simulink model "Batter_Model_02"  (Simulink 8.9)
settings: Solver=ode45  StartTime=0.0  StopTime=10.0  RelTol=1e-3  EnableMultiTasking=on
libraries: powerlib x2
settings Model: SuppressorTable=22 serialization::archive 11 0 6 0 0 0 0 0  Creator=hlopez5  LastModifiedBy=judithlopez
settings DataIOCC: SignalLoggingSaveFormat=Dataset
settings DebuggingCC: SolverPrmCheckMsg=warning  FcnCallInpInsideContextMsg=error
settings GRTTargetCC: CombineOutputUpdateFcns=on  GRTInterface=off

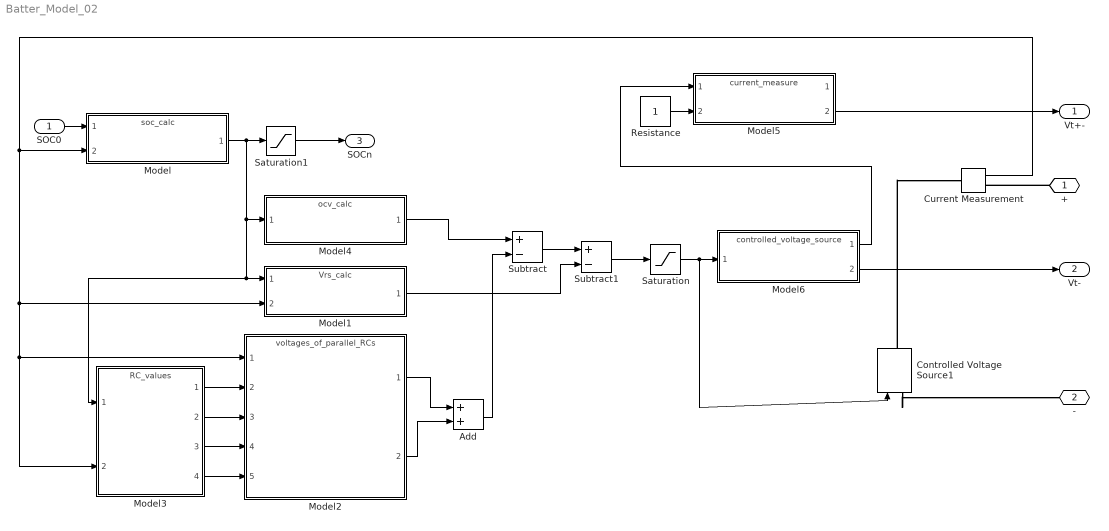
== system Batter_Model_02 ==
  SOC0 : Inport
  Add : Sum
  Controlled Voltage Source1 : powerlib/Electrical Sources/Controlled Voltage Source  Initialize=on  Source_Type=AC  Amplitude=0  Phase=0  Frequency=0  Measurements=None
  Current Measurement : powerlib/Measurements/Current Measurement  PhasorSimulation=off  OutputType=Complex  PSBequivalent=0
  Model : ModelReference  ModelNameDialog=soc_calc.mdl  SimulationMode=Normal  ModelReferenceVersion=1.2
  Model1 : ModelReference  ModelNameDialog=Vrs_calc.mdl  SimulationMode=Normal  ModelReferenceVersion=1.1
  Model2 : ModelReference  ModelNameDialog=voltages_of_parallel_RCs.mdl  SimulationMode=Normal  ModelReferenceVersion=1.3
  Model3 : ModelReference  ModelNameDialog=RC_values.mdl  SimulationMode=Normal  ModelReferenceVersion=1.3
  Model4 : ModelReference  ModelNameDialog=ocv_calc.mdl  SimulationMode=Normal  ModelReferenceVersion=1.1
  Model5 : ModelReference  ModelNameDialog=current_measure.mdl  SimulationMode=Normal  ModelReferenceVersion=1.3
  Model6 : ModelReference  ModelNameDialog=controlled_voltage_source.mdl  SimulationMode=Normal  ModelReferenceVersion=1.4
  Resistance : Constant
  Saturation : Saturate
  Saturation1 : Saturate
  Subtract : Sum  Inputs=+-
  Subtract1 : Sum  Inputs=+-
  " +" : PMIOPort  Port=1  Side=Left
  - : PMIOPort  Port=2  Side=Left
  Vt+- : Outport
  Vt- : Outport  Port=2
  SOCn : Outport  Port=3
  wires:
  Model3/1 -> Model2/2
  Model3/2 -> Model2/3
  Model3/3 -> Model2/4
  Model3/4 -> Model2/5
  Model2/1 -> Add/1
  Model2/2 -> Add/2
  Model4/1 -> Subtract/1
  Add/1 -> Subtract/2
  Subtract/1 -> Subtract1/1
  Model1/1 -> Subtract1/2
  Subtract1/1 -> Saturation/1
  SOC0/1 -> Model/1
  Model/1 -> Model3/1, Model1/1, Model4/1, Saturation1/1
  Saturation1/1 -> SOCn/1
  Current Measurement/1 -> Model3/2, Model2/1, Model1/2, Model/2
  Model5/2 -> Vt+-/1
  Saturation/1 -> Controlled Voltage Source1/1, Model6/1
  Model6/1 -> Model5/1
  Model6/2 -> Vt-/1
  Resistance/1 -> Model5/2
  connections:
  Controlled Voltage Source1/RConn1 -- Current Measurement/LConn1
  " +"/RConn1 -- Current Measurement/RConn1
  Controlled Voltage Source1/LConn1 -- -/RConn1
